simulink model "Separately_exited_DcMotor"  (R2023b)
settings: Solver=VariableStepAuto  StartTime=0.0  StopTime=0.08  MaxStep=1e-3  RelTol=1e-3
undefined symbols (not defined in the file): B, J, Kf, La, Ra, TL, Va
libraries: spsACVoltageSourceLib x1
settings Model: Creator=hp  LastModifiedBy=hp

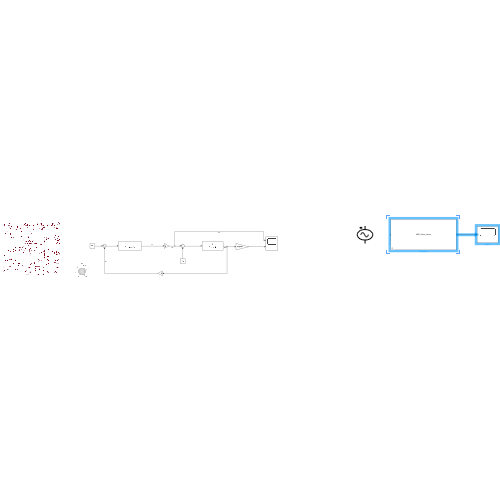
[thumbnail: Simulink's stored preview of the top-level diagram]
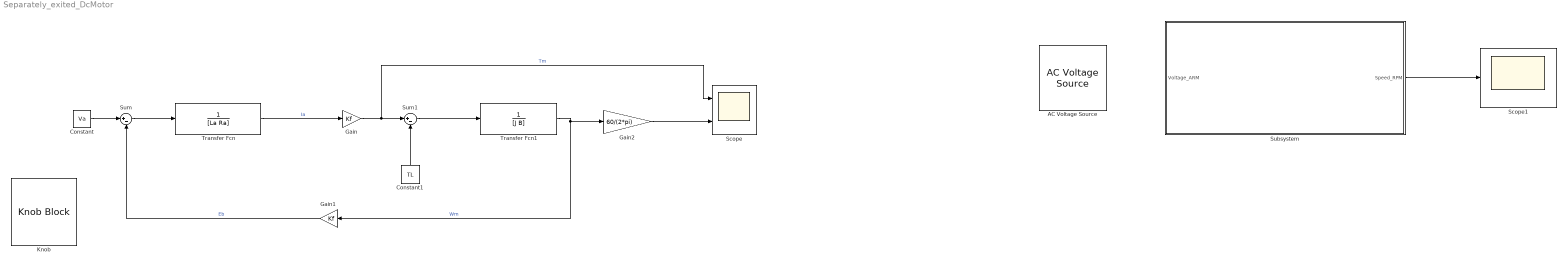
== system Separately_exited_DcMotor ==
  AC Voltage Source : spsACVoltageSourceLib/AC Voltage Source  Amplitude=100  Phase=0  Frequency=60  SampleTime=0  Measurements=None  BusType=swing  Pref=10e3  Qref=0  Qmin=-inf  Qmax=+inf
  Constant : Constant  Value=Va
  Constant1 : Constant  Value=TL
  Gain : Gain  Gain=Kf
  Gain1 : Gain  Gain=Kf
  Gain2 : Gain  Gain=60/(2*pi)
  Knob : KnobBlock  ScaleMax=220
  Scope : Scope  NumInputPorts=2
  Scope1 : Scope
  Subsystem : Subsystem  mask{Ra=0, La=0, Kf=0, J=0, B=0, TL=0}
      mask prompts: Ra "Armature Resistance"; La "Armature Inductance"; Kf "Constant"; J "Moment inertia"; B "Damping Coefficient"; TL "Load Torque"
      mask DialogControl DescGroupVar Prompt: Separately Exited Dc Motor
      mask DialogControl DescTextVar Prompt: This model reprsent to separately exited dc motor
      mask DialogControl Parameters Prompt: Parameters of model
      mask Display: disp(['SEDC_Motor_Model']);
  Sum : Sum  Inputs=|+-
  Sum1 : Sum  Inputs=|+-
  Transfer Fcn : TransferFcn  Denominator=[La Ra]
  Transfer Fcn1 : TransferFcn  Denominator=[J B]
  wires:
  Sum/1 -> Transfer Fcn/1
  Transfer Fcn/1 -> Gain/1  "Ia"
  Gain/1 -> Scope/1, Sum1/1  "Tm"
  Sum1/1 -> Transfer Fcn1/1
  Transfer Fcn1/1 -> Gain2/1, Gain1/1  "Wm"
  Gain1/1 -> Sum/2  "Eb"
  Gain2/1 -> Scope/2
  Constant1/1 -> Sum1/2
  Constant/1 -> Sum/1
  Subsystem/1(Speed_RPM) -> Scope1/1

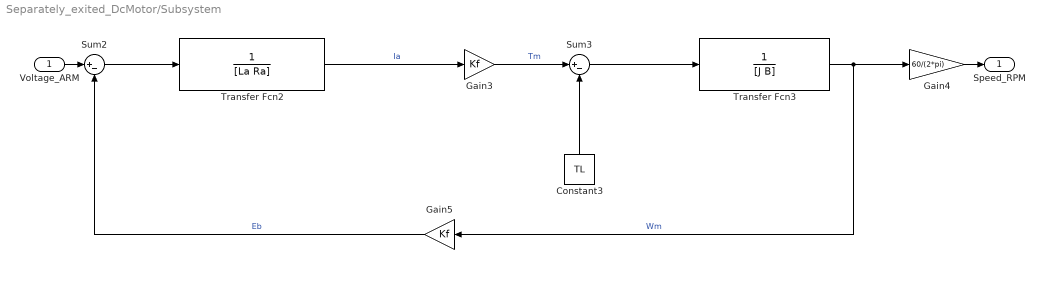
== system Separately_exited_DcMotor/Subsystem ==
  Voltage_ARM : Inport
  Constant3 : Constant  Value=TL
  Gain3 : Gain  Gain=Kf
  Gain4 : Gain  Gain=60/(2*pi)
  Gain5 : Gain  Gain=Kf
  Sum2 : Sum  Inputs=|+-
  Sum3 : Sum  Inputs=|+-
  Transfer Fcn2 : TransferFcn  Denominator=[La Ra]
  Transfer Fcn3 : TransferFcn  Denominator=[J B]
  Speed_RPM : Outport
  wires:
  Gain5/1 -> Sum2/2  "Eb"
  Constant3/1 -> Sum3/2
  Gain3/1 -> Sum3/1  "Tm"
  Voltage_ARM/1 -> Sum2/1
  Transfer Fcn2/1 -> Gain3/1  "Ia"
  Transfer Fcn3/1 -> Gain5/1, Gain4/1  "Wm"
  Sum3/1 -> Transfer Fcn3/1
  Sum2/1 -> Transfer Fcn2/1
  Gain4/1 -> Speed_RPM/1
